simulink model "pidControllerAltitude2023aSubsystems"  (R2023a)
settings: Solver=VariableStepAuto  StartTime=0.0  StopTime=10.0  RelTol=1e-3
settings Model: Creator=Ditte  LastModifiedBy=Ditte

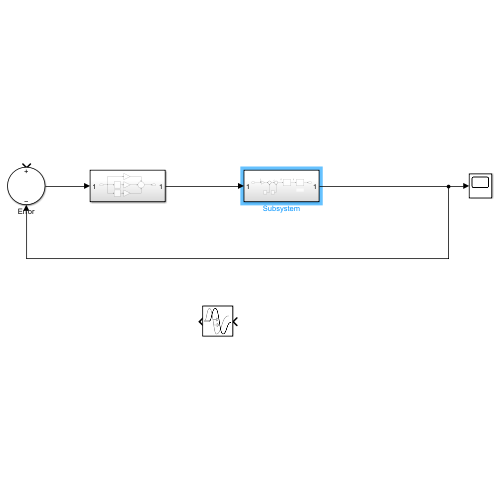
[thumbnail: Simulink's stored preview of the top-level diagram]
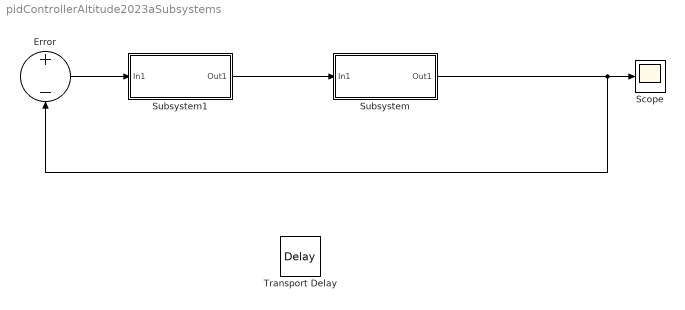
== system pidControllerAltitude2023aSubsystems ==
  Error : Sum  Inputs=+-
  Scope : Scope
  Subsystem : Subsystem
  Subsystem1 : Subsystem
  Transport Delay : TransportDelay  DelayTime=0.0000025
  wires:
  Error/1 -> Subsystem1/1(In1)
  Subsystem1/1(Out1) -> Subsystem/1(In1)
  Subsystem/1(Out1) -> Error/2, Scope/1

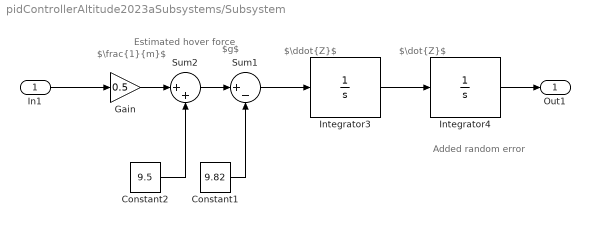
== system pidControllerAltitude2023aSubsystems/Subsystem ==
  note: $\ddot{Z}$
  note: $g$
  note: $\dot{Z}$
  note: Estimated
      | hover force
  note: Added random
      | error
  note: $\frac{1}{m}$
  In1 : Inport
  Constant1 : Constant  Value=9.82
  Constant2 : Constant  Value=9.5
  Gain : Gain  Gain=0.5
  Integrator3 : Integrator
  Integrator4 : Integrator  LimitOutput=on  LowerSaturationLimit=0
  Sum1 : Sum  Inputs=|+-
  Sum2 : Sum  Inputs=|++
  Out1 : Outport
  wires:
  Integrator4/1 -> Out1/1
  Constant2/1 -> Sum2/2
  Constant1/1 -> Sum1/2
  Gain/1 -> Sum2/1
  Integrator3/1 -> Integrator4/1
  In1/1 -> Gain/1
  Sum2/1 -> Sum1/1
  Sum1/1 -> Integrator3/1

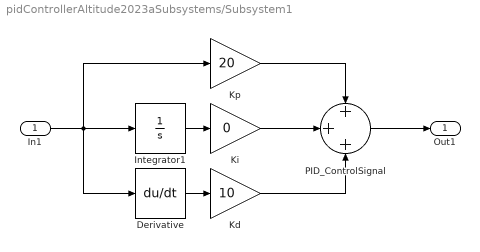
== system pidControllerAltitude2023aSubsystems/Subsystem1 ==
  In1 : Inport
  Derivative : Derivative
  Integrator1 : Integrator
  Kd : Gain  Gain=10
  Ki : Gain  Gain=0
  Kp : Gain  Gain=20
  PID_ControlSignal : Sum  Inputs=+++
  Out1 : Outport
  wires:
  Ki/1 -> PID_ControlSignal/2
  Kp/1 -> PID_ControlSignal/1
  In1/1 -> Derivative/1, Integrator1/1, Kp/1
  PID_ControlSignal/1 -> Out1/1
  Integrator1/1 -> Ki/1
  Derivative/1 -> Kd/1
  Kd/1 -> PID_ControlSignal/3
